simulink model "Lab_1_170747"  (R2019a)
settings: Solver=ode2  StartTime=0.0  StopTime=100  RelTol=1e-3  EnableMultiTasking=on
settings Model: Creator=shivali  LastModifiedBy=singh
settings DataIOCC: ReturnWorkspaceOutputs=off
settings OptimizationCC: LifeSpan=inf
settings DebuggingCC: SFUnexpectedBacktrackingDiag=warning  SFNoUnconditionalDefaultTransitionDiag=warning  ArithmeticOperatorsInVariantConditions=warning
settings SFSimCC: SimUseLocalCustomCode=off
settings RTWCC: RTWUseLocalCustomCode=off
settings CodeAppCC: StateflowObjectComments=on
settings GRTTargetCC: TargetLangStandard=C89/C90 (ANSI)  GeneratePreprocessorConditionals=Disable all
settings ConfigComp: CovMetricSettings=dw  CovHtmlReporting=on  CovSaveCumulativeToWorkspaceVar=on  CovSaveSingleToWorkspaceVar=on  CovExternalEMLEnable=off

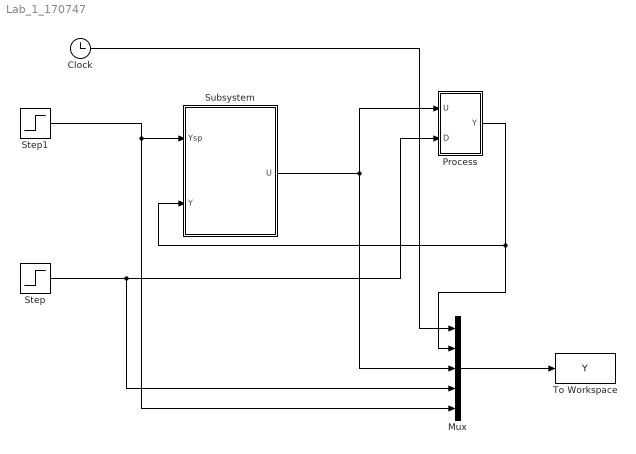
== system Lab_1_170747 ==
  Clock : Clock
  Mux : Mux  Inputs=5
  Process : Subsystem
  Step : Step  After=0  SampleTime=0
  Step1 : Step  SampleTime=.1
  Subsystem : Subsystem  mask{Kc=-0.3700, Ti=8, Td=1}
      mask prompts: Kc "Proportional Gain"; Ti "Integral Time"; Td "Derivative Time"
  To Workspace : ToWorkspace  VariableName=Y  SampleTime=-1
  wires:
  Subsystem/1(U) -> Process/1(U), Mux/3
  Step/1 -> Mux/4, Process/2(D)
  Step1/1 -> Mux/5, Subsystem/1(Ysp)
  Process/1(Y) -> Mux/2, Subsystem/2(Y)
  Clock/1 -> Mux/1
  Mux/1 -> To Workspace/1

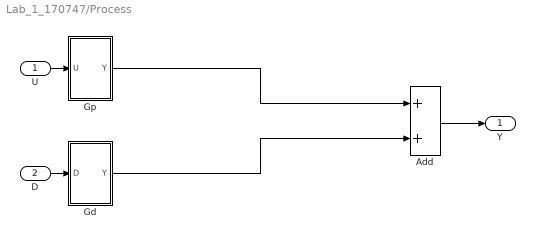
== system Lab_1_170747/Process ==
  U : Inport
  D : Inport  Port=2
  Add : Sum
  Gd : Subsystem
  Gp : Subsystem
  Y : Outport
  wires:
  Gp/1(Y) -> Add/1
  Add/1 -> Y/1
  U/1 -> Gp/1(U)
  D/1 -> Gd/1(D)
  Gd/1(Y) -> Add/2

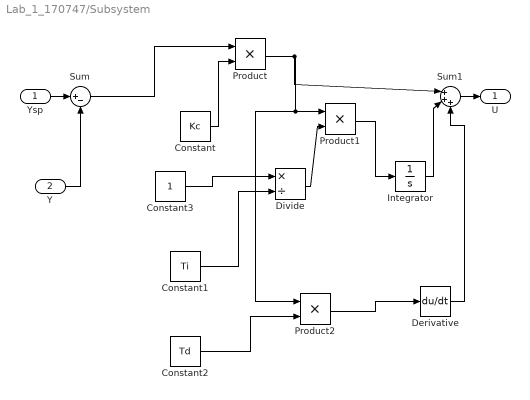
== system Lab_1_170747/Subsystem ==
  Ysp : Inport
  Y : Inport  Port=2
  Constant : Constant  Value=Kc
  Constant1 : Constant  Value=Ti
  Constant2 : Constant  Value=Td
  Constant3 : Constant
  Derivative : Derivative
  Divide : Product  Inputs=*/
  Integrator : Integrator
  Product : Product
  Product1 : Product
  Product2 : Product
  Sum : Sum  Inputs=|+-
  Sum1 : Sum  Inputs=|+++
  U : Outport
  wires:
  Product1/1 -> Integrator/1
  Divide/1 -> Product1/2
  Constant2/1 -> Product2/2
  Integrator/1 -> Sum1/2
  Product/1 -> Sum1/1, Product1/1, Product2/1
  Sum1/1 -> U/1
  Sum/1 -> Product/1
  Constant/1 -> Product/2
  Product2/1 -> Derivative/1
  Derivative/1 -> Sum1/3
  Constant1/1 -> Divide/2
  Constant3/1 -> Divide/1
  Ysp/1 -> Sum/1
  Y/1 -> Sum/2

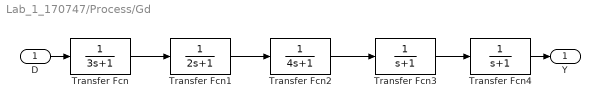
== system Lab_1_170747/Process/Gd ==
  D : Inport
  Transfer Fcn : TransferFcn  Denominator=[3 1]
  Transfer Fcn1 : TransferFcn  Denominator=[2 1]
  Transfer Fcn2 : TransferFcn  Denominator=[4 1]
  Transfer Fcn3 : TransferFcn  Denominator=[1 1]
  Transfer Fcn4 : TransferFcn  Denominator=[1 1]
  Y : Outport
  wires:
  Transfer Fcn1/1 -> Transfer Fcn2/1
  D/1 -> Transfer Fcn/1
  Transfer Fcn4/1 -> Y/1
  Transfer Fcn3/1 -> Transfer Fcn4/1
  Transfer Fcn/1 -> Transfer Fcn1/1
  Transfer Fcn2/1 -> Transfer Fcn3/1

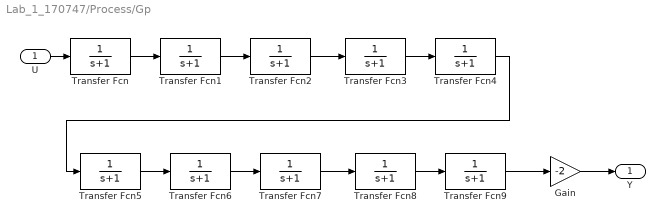
== system Lab_1_170747/Process/Gp ==
  U : Inport
  Gain : Gain  Gain=-2
  Transfer Fcn{,1..9} (10 alike) : TransferFcn  Denominator=[1 1]
  Y : Outport
  wires:
  Transfer Fcn1/1 -> Transfer Fcn2/1
  Transfer Fcn2/1 -> Transfer Fcn3/1
  Transfer Fcn/1 -> Transfer Fcn1/1
  Transfer Fcn4/1 -> Transfer Fcn5/1
  Transfer Fcn3/1 -> Transfer Fcn4/1
  U/1 -> Transfer Fcn/1
  Transfer Fcn7/1 -> Transfer Fcn8/1
  Transfer Fcn5/1 -> Transfer Fcn6/1
  Transfer Fcn8/1 -> Transfer Fcn9/1
  Transfer Fcn6/1 -> Transfer Fcn7/1
  Transfer Fcn9/1 -> Gain/1
  Gain/1 -> Y/1
